simulink model "project"  (R2021a)
settings: Solver=VariableStepAuto  StartTime=0.0  StopTime=40  RelTol=1e-3
undefined symbols (not defined in the file or in its folder): ZigBee
libraries: truetime x13, fuzblock x1
settings Model: EnablePacing=on  Creator=Luigi Pio  LastModifiedBy=Luigi Pio

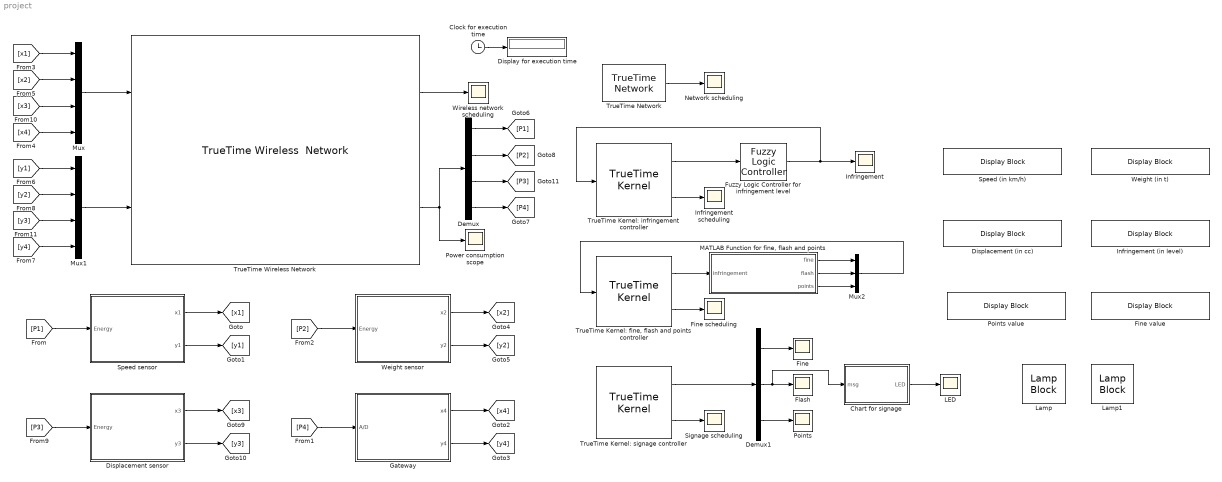
== system project ==
  "Chart for signage " : Stateflow chart  TreatAsAtomicUnit=on
  Clock for execution time : Clock
  Demux : Demux
  Demux1 : Demux  Outputs=3
  Displacement (in cc) : DisplayBlock  LabelPosition=Hide  Format=Integer  Transparency=1
  Displacement sensor : Subsystem
  Display for execution time : Display
  Fine : Scope
  Fine scheduling : Scope
  Fine value : DisplayBlock  LabelPosition=Hide  Transparency=1
  Flash : Scope
  Fuzzy Logic Controller for infringement level : fuzblock/Fuzzy Logic  Controller  FIS='controller.fis'  OutputSampleNumber=101  DataType=double  FuzzifiedInputs=off  RuleFiringStrengths=off  RuleOutputs=off  AggregatedOutputs=off  SimulateUsing=Interpreted execution  OutOfRangeInputValueMessage=warning  NoRuleFiredMessage=warning  EmptyOutputFuzzySetMessage=warning
  Gateway : Subsystem
  Infringement : Scope
  Infringement scheduling : Scope
  Infringement (in level) : DisplayBlock  LabelPosition=Hide  Transparency=1
  LED : Scope
  Lamp : LampBlock  LabelPosition=Hide
  Lamp1 : LampBlock  LabelPosition=Hide
  "MATLAB Function for fine, flash and points" : MATLAB Function  TreatAsAtomicUnit=on
  Mux : Mux
  Mux1 : Mux
  Mux2 : Mux  Inputs=3
  Network scheduling : Scope
  Points : Scope
  Points value : DisplayBlock  LabelPosition=Hide  Transparency=1
  Power consumption scope : Scope
  Signage scheduling : Scope
  Speed (in km/h) : DisplayBlock  LabelPosition=Hide  Format=Integer  Transparency=1
  Speed sensor : Subsystem
  "TrueTime Kernel: fine, flash and points controller" : truetime/TrueTime Kernel  sfun=fineFlashPointsController_init  args=[]  ninputsoutputs=[3 1]  ntriggers=0  trigtype=falling  nwnodenbr=[2 3]  clockoffsetdrift=[0 0]  schedoutput=on  battery=off  poweroutput=off  label=2: 3
  TrueTime Kernel: infringement controller : truetime/TrueTime Kernel  sfun=infringementController_init  args=[]  ninputsoutputs=[1 3]  ntriggers=0  trigtype=falling  nwnodenbr=[2 2]  clockoffsetdrift=[0 0]  schedoutput=on  battery=off  poweroutput=off  label=2: 2
  TrueTime Kernel: signage controller : truetime/TrueTime Kernel  sfun=signageController_init  args=[]  ninputsoutputs=[0 3]  ntriggers=0  trigtype=falling  nwnodenbr=[2 4]  clockoffsetdrift=[0 0]  schedoutput=on  battery=off  poweroutput=off  label=2: 4
  "TrueTime Network " : truetime/TrueTime Network  nwtype=CSMA/CD (Ethernet)  nwnbr=2  nnodes=4  rate=10000000  minsize=512  lossprob=0  seed=0  bandwidths=[0.5 0.5]  slotsize=512  schedule=[1 1 2]  memsize=80000  buftype=Common buffer  overflow=Retransmit  dynSchedule=0  miniSlotSize=0  NIT=0  QSortMode=FIFO  sync=0  irtSchedule=0  nrtLength=0  nodeGraph=0  scheduleoutput=on
  "TrueTime Wireless Network " : truetime/TrueTime Wireless  Network  nwtype=802.15.4 (ZigBee)  nwnbr=1  nnodes=4  rate=800000  minsize=272  transpower=20  threshold=-48  use_pathloss_function=default  pathloss=3.5  acktimeout=0.00004  retrylimit=5  error_threshold=0.03  lossprob=0  seed=0  scheduleoutput=on  poweroutput=on
  Weight (in t) : DisplayBlock  LabelPosition=Hide  Format=Integer  Transparency=1
  Weight sensor : Subsystem
  Wireless network scheduling : Scope
  wires:
  [P1] -> Speed sensor/1(Energy)
  Speed sensor/1(x1) -> [x1]
  Speed sensor/2(y1) -> [y1]
  [P4] -> Gateway/1(A/D)
  Gateway/1(x4) -> [x4]
  Gateway/2(y4) -> [y4]
  [P2] -> Weight sensor/1(Energy)
  Weight sensor/1(x2) -> [x2]
  Weight sensor/2(y2) -> [y2]
  Mux/1 -> "TrueTime Wireless Network "/1
  Mux1/1 -> "TrueTime Wireless Network "/2
  [x1] -> Mux/1
  [x2] -> Mux/2
  [y2] -> Mux1/2
  [y1] -> Mux1/1
  "TrueTime Wireless Network "/1 -> Wireless network scheduling/1
  "TrueTime Wireless Network "/2 -> Demux/1, Power consumption scope/1
  Demux/1 -> [P1]
  Demux/2 -> [P2]
  TrueTime Kernel: signage controller/1 -> Demux1/1
  Demux1/1 -> Fine/1
  Demux1/2 -> Flash/1, "Chart for signage "/1(msg)
  Demux1/3 -> Points/1
  TrueTime Kernel: signage controller/2 -> Signage scheduling/1
  "Chart for signage "/1(LED) -> LED/1
  "TrueTime Kernel: fine, flash and points controller"/1 -> "MATLAB Function for fine, flash and points"/1(infringement)
  "MATLAB Function for fine, flash and points"/1(fine) -> Mux2/1
  Mux2/1 -> "TrueTime Kernel: fine, flash and points controller"/1
  "TrueTime Kernel: fine, flash and points controller"/2 -> Fine scheduling/1
  TrueTime Kernel: infringement controller/1 -> Fuzzy Logic Controller for infringement level/1
  Fuzzy Logic Controller for infringement level/1 -> TrueTime Kernel: infringement controller/1, Infringement/1
  TrueTime Kernel: infringement controller/2 -> Infringement scheduling/1
  "TrueTime Network "/1 -> Network scheduling/1
  "MATLAB Function for fine, flash and points"/2(flash) -> Mux2/2
  "MATLAB Function for fine, flash and points"/3(points) -> Mux2/3
  Displacement sensor/2(y3) -> [y3]
  Displacement sensor/1(x3) -> [x3]
  [P3] -> Displacement sensor/1(Energy)
  [x3] -> Mux/3
  [y3] -> Mux1/3
  Demux/3 -> [P3]
  [x4] -> Mux/4
  [y4] -> Mux1/4
  Demux/4 -> [P4]
  Clock for execution time/1 -> Display for execution time/1

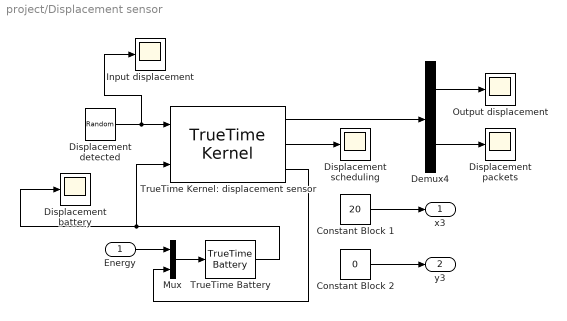
== system project/Displacement sensor ==
  Energy : Inport  Interpolate=off
  Constant Block 1 : Constant  Value=20
  Constant Block 2 : Constant  Value=0
  Demux4 : Demux  Outputs=2
  Displacement scheduling : Scope
  Displacement battery : Scope
  Displacement detected : UniformRandomNumber  Minimum=0  Maximum=3000  Seed=5  SampleTime=2
  Displacement packets : Scope
  Input displacement : Scope
  Mux : Mux  Inputs=2
  Output displacement : Scope
  "TrueTime Battery " : truetime/TrueTime Battery  energy=5
  TrueTime Kernel: displacement sensor : truetime/TrueTime Kernel  sfun=displacementSensor_init  args=[]  ninputsoutputs=[1 2]  ntriggers=0  trigtype=falling  nwnodenbr=[1 3]  clockoffsetdrift=[0 0]  schedoutput=on  battery=on  poweroutput=on  label=1: 3
  x3 : Outport
  y3 : Outport  Port=2
  wires:
  Energy/1 -> Mux/1
  TrueTime Kernel: displacement sensor/2 -> Displacement scheduling/1
  Mux/1 -> "TrueTime Battery "/1
  Displacement detected/1 -> TrueTime Kernel: displacement sensor/1, Input displacement/1
  TrueTime Kernel: displacement sensor/3 -> Mux/2
  Constant Block 2/1 -> y3/1
  Constant Block 1/1 -> x3/1
  TrueTime Kernel: displacement sensor/1 -> Demux4/1
  Demux4/2 -> Displacement packets/1
  Demux4/1 -> Output displacement/1
  "TrueTime Battery "/1 -> Displacement battery/1, TrueTime Kernel: displacement sensor/2

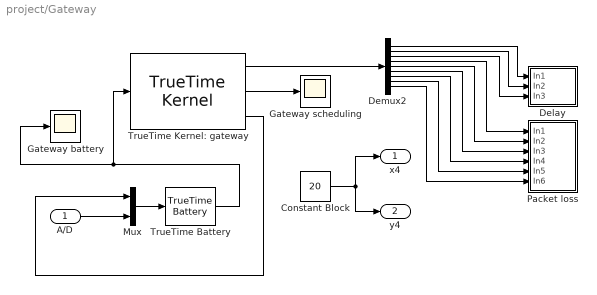
== system project/Gateway ==
  A/D : Inport  Interpolate=off
  Constant Block : Constant  Value=20
  "Delay " : Subsystem
  Demux2 : Demux  Outputs=9
  Gateway battery : Scope
  Gateway scheduling : Scope
  Mux : Mux  Inputs=2
  Packet loss : Subsystem
  "TrueTime Battery " : truetime/TrueTime Battery  energy=5
  TrueTime Kernel: gateway : truetime/TrueTime Kernel  sfun=gateway_init  args=[]  ninputsoutputs=[0 9]  ntriggers=0  trigtype=falling  nwnodenbr=[1 4; 2 1]  clockoffsetdrift=[0 0]  schedoutput=on  battery=on  poweroutput=on  label=1: 4\n2: 1
  x4 : Outport
  y4 : Outport  Port=2
  wires:
  A/D/1 -> Mux/2
  TrueTime Kernel: gateway/2 -> Gateway scheduling/1
  Mux/1 -> "TrueTime Battery "/1
  TrueTime Kernel: gateway/3 -> Mux/1
  Demux2/2 -> "Delay "/2(In2)
  Demux2/1 -> "Delay "/1(In1)
  TrueTime Kernel: gateway/1 -> Demux2/1
  Demux2/3 -> "Delay "/3(In3)
  Demux2/4 -> Packet loss/1(In1)
  Demux2/5 -> Packet loss/2(In2)
  Demux2/6 -> Packet loss/3(In3)
  Demux2/7 -> Packet loss/4(In4)
  Demux2/8 -> Packet loss/5(In5)
  Demux2/9 -> Packet loss/6(In6)
  "TrueTime Battery "/1 -> Gateway battery/1, TrueTime Kernel: gateway/1
  Constant Block/1 -> y4/1, x4/1

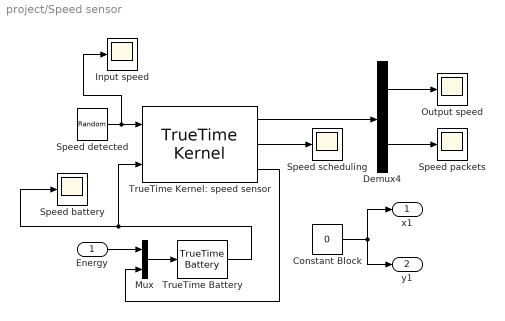
== system project/Speed sensor ==
  Energy : Inport  Interpolate=off
  Constant Block : Constant  Value=0
  Demux4 : Demux  Outputs=2
  Input speed : Scope
  Mux : Mux  Inputs=2
  Output speed : Scope
  Speed battery : Scope
  Speed detected : UniformRandomNumber  Minimum=0  Maximum=220  Seed=5  SampleTime=2
  Speed packets : Scope
  Speed scheduling : Scope
  "TrueTime Battery " : truetime/TrueTime Battery  energy=5
  TrueTime Kernel: speed sensor : truetime/TrueTime Kernel  sfun=speedSensor_init  args=[]  ninputsoutputs=[1 2]  ntriggers=0  trigtype=falling  nwnodenbr=[1 1]  clockoffsetdrift=[0 0]  schedoutput=on  battery=on  poweroutput=on  label=1: 1
  x1 : Outport
  y1 : Outport  Port=2
  wires:
  Energy/1 -> Mux/1
  TrueTime Kernel: speed sensor/2 -> Speed scheduling/1
  Mux/1 -> "TrueTime Battery "/1
  Speed detected/1 -> Input speed/1, TrueTime Kernel: speed sensor/1
  TrueTime Kernel: speed sensor/3 -> Mux/2
  Demux4/2 -> Speed packets/1
  Demux4/1 -> Output speed/1
  TrueTime Kernel: speed sensor/1 -> Demux4/1
  "TrueTime Battery "/1 -> TrueTime Kernel: speed sensor/2, Speed battery/1
  Constant Block/1 -> y1/1, x1/1

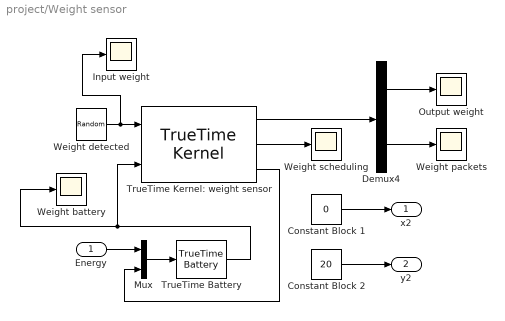
== system project/Weight sensor ==
  Energy : Inport  Interpolate=off
  Constant Block 1 : Constant  Value=0
  Constant Block 2 : Constant  Value=20
  Demux4 : Demux  Outputs=2
  Input weight : Scope
  Mux : Mux  Inputs=2
  Output weight : Scope
  "TrueTime Battery " : truetime/TrueTime Battery  energy=5
  TrueTime Kernel: weight sensor : truetime/TrueTime Kernel  sfun=weightSensor_init  args=[]  ninputsoutputs=[1 2]  ntriggers=0  trigtype=falling  nwnodenbr=[1 2]  clockoffsetdrift=[0 0]  schedoutput=on  battery=on  poweroutput=on  label=1: 2
  Weight battery : Scope
  Weight detected : UniformRandomNumber  Minimum=0  Maximum=20  Seed=5  SampleTime=2
  Weight packets : Scope
  Weight scheduling : Scope
  x2 : Outport
  y2 : Outport  Port=2
  wires:
  Energy/1 -> Mux/1
  TrueTime Kernel: weight sensor/2 -> Weight scheduling/1
  Mux/1 -> "TrueTime Battery "/1
  Weight detected/1 -> Input weight/1, TrueTime Kernel: weight sensor/1
  TrueTime Kernel: weight sensor/3 -> Mux/2
  Constant Block 2/1 -> y2/1
  Constant Block 1/1 -> x2/1
  TrueTime Kernel: weight sensor/1 -> Demux4/1
  Demux4/2 -> Weight packets/1
  Demux4/1 -> Output weight/1
  "TrueTime Battery "/1 -> Weight battery/1, TrueTime Kernel: weight sensor/2

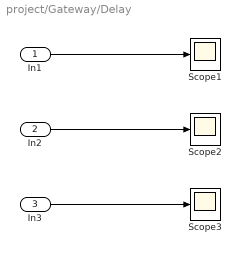
== system project/Gateway/Delay  ==
  In1 : Inport
  In2 : Inport  Port=2
  In3 : Inport  Port=3
  Scope1 : Scope
  Scope2 : Scope
  Scope3 : Scope
  wires:
  In3/1 -> Scope3/1
  In2/1 -> Scope2/1
  In1/1 -> Scope1/1

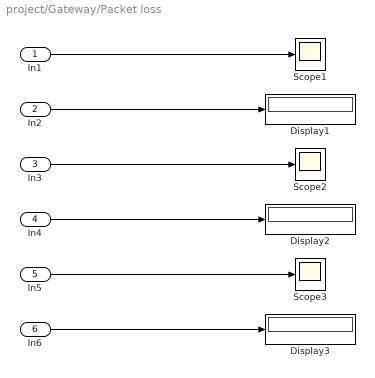
== system project/Gateway/Packet loss ==
  In1 : Inport
  In2 : Inport  Port=2
  In3 : Inport  Port=3
  In4 : Inport  Port=4
  In5 : Inport  Port=5
  In6 : Inport  Port=6
  Display1 : Display
  Display2 : Display
  Display3 : Display
  Scope1 : Scope
  Scope2 : Scope
  Scope3 : Scope
  wires:
  In5/1 -> Scope3/1
  In2/1 -> Display1/1
  In6/1 -> Display3/1
  In4/1 -> Display2/1
  In1/1 -> Scope1/1
  In3/1 -> Scope2/1

== matlab function project/MATLAB Function for fine, flash and points ==
  data: infringement input; fine output; flash output; points output
function [fine, flash, points] = fcn(infringement)
fine = 0;
flash = 0;
points = 0;

% Caso "No_Circulate"
if infringement == 1
    fine = 103;
    flash = 1;
    points = -2;

% Caso "Low"
elseif infringement == 2
    fine = 105;
    flash = 1;
    points = 0;

% Caso "Medium"
elseif infringement == 3
    fine = 421;
    flash = 1;
    points = -3;

% Caso "High"
elseif infringement == 4
    fine = 1318;
    flash = 1;
    points = -6;

% Caso "Very_High"
elseif infringement == 5
    fine = 2054;
    flash = 1;
    points = -10;
end
end

== stateflow chart project/Chart for signage  ==
  state Signage
    state Initialization
      entry:LED=0;
    state OnOff
      state On
        entry:LED=1;
      state Off
        entry:LED=2;
      (default) -> On
      On -> Off : [after(0.25,sec)]
      Off -> On : [after(0.25,sec)]
    (default) -> Initialization
    Initialization -> OnOff : [msg == 1]
    OnOff -> Initialization : [msg == 0]
  data: msg input; LED output
